simulink model "jifenzhuangtaiguanceqi"  (R2022b)
settings: Solver=VariableStepAuto  StartTime=0.0  StopTime=20  RelTol=1e-3
settings Model: Creator=HONOR  LastModifiedBy=acer
settings DebuggingCC: UnconnectedInputMsg=warning  UnconnectedOutputMsg=warning  UnconnectedLineMsg=warning
settings ModelReferenceCC: EnableRefExpFcnMdlSchedulingChecks=on
settings RTWCC: DLArmComputeVersion=19.05

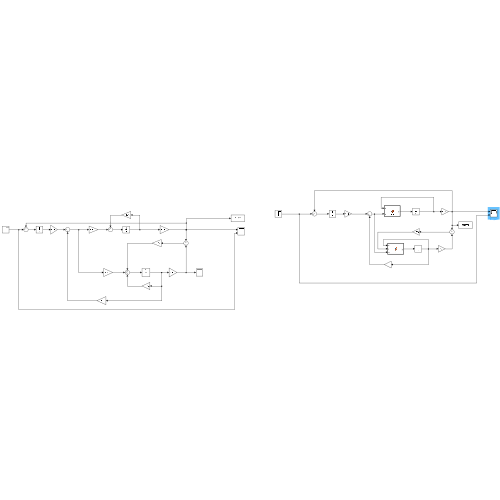
[thumbnail: Simulink's stored preview of the top-level diagram]
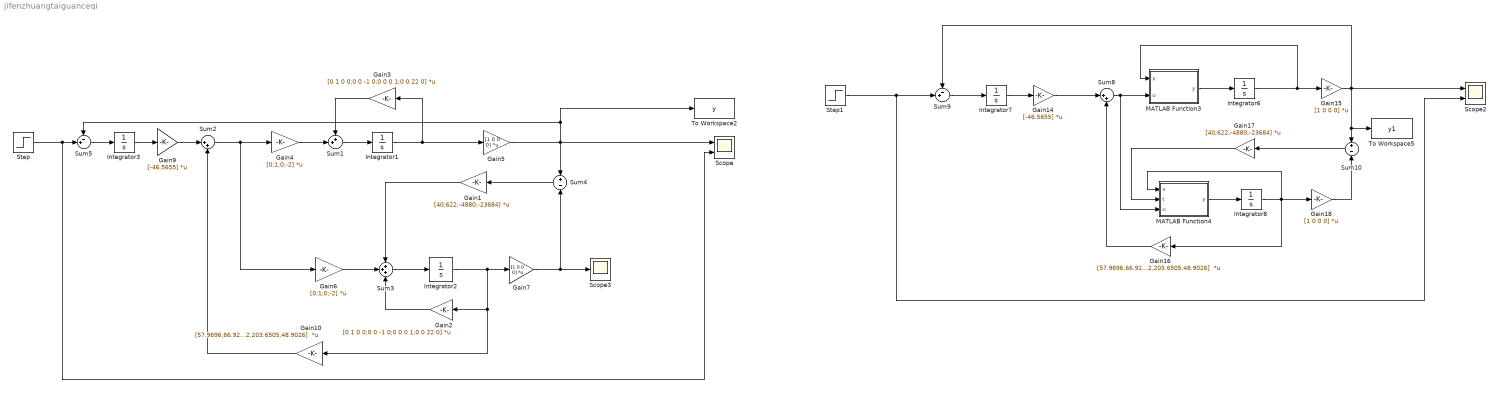
== system jifenzhuangtaiguanceqi ==
  Gain1 : Gain  Gain=[40;622;-4880;-23684]  Multiplication=Matrix(K*u)
  Gain10 : Gain  Gain=[57.9696,66.9252,203.6505,48.9026]  Multiplication=Matrix(K*u)
  Gain14 : Gain  Gain=[-46.5655]  Multiplication=Matrix(K*u)
  Gain{5,7,15,18} (4 alike) : Gain  Gain=[1 0 0 0]  Multiplication=Matrix(K*u)
  Gain16 : Gain  Gain=[57.9696,66.9252,203.6505,48.9026]  Multiplication=Matrix(K*u)
  Gain17 : Gain  Gain=[40;622;-4880;-23684]  Multiplication=Matrix(K*u)
  Gain2 : Gain  Gain=[0 1 0 0;0 0 -1 0;0 0 0 1;0 0 22 0]  Multiplication=Matrix(K*u)
  Gain3 : Gain  Gain=[0 1 0 0;0 0 -1 0;0 0 0 1;0 0 22 0]  Multiplication=Matrix(K*u)
  Gain4 : Gain  Gain=[0;1;0;-2]  Multiplication=Matrix(K*u)
  Gain6 : Gain  Gain=[0;1;0;-2]  Multiplication=Matrix(K*u)
  Gain9 : Gain  Gain=[-46.5655]  Multiplication=Matrix(K*u)
  Integrator1 : Integrator  InitialCondition=[0,0,0.1,0]
  Integrator2 : Integrator  InitialCondition=[0,0,0,0]
  Integrator3 : Integrator  InitialCondition=[0]
  Integrator6 : Integrator  InitialCondition=[0,0,0.1,0]
  Integrator7 : Integrator  InitialCondition=[0]
  Integrator8 : Integrator  InitialCondition=[0,0,0,0]
  MATLAB Function3 : MATLAB Function  TreatAsAtomicUnit=on
  MATLAB Function4 : MATLAB Function  TreatAsAtomicUnit=on
  Scope : Scope  NumInputPorts=2
  Scope2 : Scope  NumInputPorts=2
  Scope3 : Scope
  Step : Step  SampleTime=0
  Step1 : Step  SampleTime=0
  Sum1 : Sum  Inputs=++|
  Sum10 : Sum  Inputs=+-
  Sum2 : Sum  Inputs=|++
  Sum3 : Sum  Inputs=+++
  Sum4 : Sum  Inputs=+|-
  Sum5 : Sum  Inputs=-+|
  Sum8 : Sum  Inputs=|++
  Sum9 : Sum  Inputs=-+|
  To Workspace2 : ToWorkspace  VariableName=y  SaveFormat=Structure With Time  SampleTime=-1
  To Workspace5 : ToWorkspace  VariableName=y1  SaveFormat=Structure With Time  SampleTime=-1
  wires:
  Step/1 -> Scope/2, Sum5/2
  Integrator1/1 -> Gain5/1, Gain3/1
  Gain7/1 -> Scope3/1, Sum4/2
  Integrator3/1 -> Gain9/1
  Integrator2/1 -> Gain7/1, Gain10/1, Gain2/1
  Gain9/1 -> Sum2/1
  Gain3/1 -> Sum1/1
  Sum4/1 -> Gain1/1
  Sum2/1 -> Gain6/1, Gain4/1
  Gain4/1 -> Sum1/2
  Sum5/1 -> Integrator3/1
  Sum1/1 -> Integrator1/1
  Sum3/1 -> Integrator2/1
  Gain5/1 -> Scope/1, To Workspace2/1, Sum5/1, Sum4/1
  Gain10/1 -> Sum2/2
  Step1/1 -> Scope2/2, Sum9/2
  Integrator7/1 -> Gain14/1
  Gain16/1 -> Sum8/2
  Sum8/1 -> MATLAB Function4/3(u), MATLAB Function3/2(u)
  Sum9/1 -> Integrator7/1
  MATLAB Function3/1(y) -> Integrator6/1
  Gain14/1 -> Sum8/1
  Integrator6/1 -> MATLAB Function3/1(x), Gain15/1
  Gain15/1 -> Sum10/1, To Workspace5/1, Sum9/1, Scope2/1
  Sum10/1 -> Gain17/1
  MATLAB Function4/1(y) -> Integrator8/1
  Integrator8/1 -> Gain16/1, MATLAB Function4/1(x), Gain18/1
  Gain18/1 -> Sum10/2
  Gain17/1 -> MATLAB Function4/2(t)
  Gain6/1 -> Sum3/2
  Gain2/1 -> Sum3/3
  Gain1/1 -> Sum3/1

== matlab function jifenzhuangtaiguanceqi/MATLAB Function4 ==
  data: x input; t input; u input; y output
function y = fcn(x, t, u)
M=1;
m=0.1;
l=0.5;
g=10;
Dx3=x(4)+t(3);
Dx4=(u*cos(x(3))-(M+m)*g*sin(x(3))+m*l*sin(x(3))*cos(x(3)*x(4)))/(m*l*cos(x(3))*cos(x(3))-(M+m)*l)+t(4);
Dx1=x(2)+t(1);
Dx2=((u+m*l*sin(x(3)*x(4)*x(4))-m*g*cos(x(3))*sin(x(3)))/(M+m-m*cos(x(3))*cos(x(3))))+t(2);
y=[Dx1;Dx2;Dx3;Dx4];

== matlab function jifenzhuangtaiguanceqi/MATLAB Function3 ==
  data: x input; u input; y output
function y = fcn(x, u)
M=1;
m=0.1;
l=0.5;
g=10;
Dx3=x(4);
Dx4=(u*cos(x(3))-(M+m)*g*sin(x(3))+m*l*sin(x(3))*cos(x(3)*x(4)))/(m*l*cos(x(3))*cos(x(3))-(M+m)*l);
Dx1=x(2);
Dx2=((u+m*l*sin(x(3)*x(4)*x(4))-m*g*cos(x(3))*sin(x(3)))/(M+m-m*cos(x(3))*cos(x(3))));
y=[Dx1;Dx2;Dx3;Dx4];
